simulink model "AION_IDS_SPEEDGOAT"  (R2021a)
settings: configuration reference "AION_IDS_Speedgoat" (kept outside this file)
undefined symbols (not defined in the file): ADCU_SCU_CYCLE_TIME, AutoTrqWhlReq_test, BeamReq_test, BodyCtrlReq_test, BrakeReq_test, C, CONTROL_CYCLE_TIME, GearLvlReq_test, GearLvlReqVD_test, HornRingReq_test, LatCtrlReq_test, LngCtrlReq_test, SCU_ADCU_CYCLE_TIME, SteerAngReq_test, SteerWhlTorqReq_test, TurnLightReq_test
libraries: canmsglib x21, speedgoatlib_IO612 x8, simulink x1
(part 1 of 2)
settings Model: DataDictionary=AION_IDS.sldd  SimulationMode=external  ExtModeBatchMode=on  ExtModeTrigType=signal  Creator=xinrui  LastModifiedBy=Administrator
settings ConfigSetRef: SourceName=AION_IDS_Speedgoat

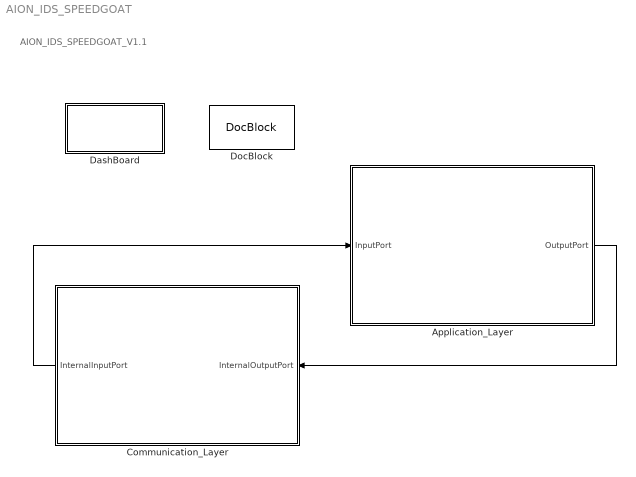
== system AION_IDS_SPEEDGOAT ==
  note: AION_IDS_SPEEDGOAT_V1.1
  Application_Layer : Subsystem
  Communication_Layer : Subsystem
  DashBoard : Subsystem
  DocBlock : simulink/Model-Wide Utilities/DocBlock  DocumentType=HTML  mask(DocBlock){}
      mask Display:
      | plot([.8 0 0 1 1 .8 .8 1],[1 1 0 0 .8 1 .8 .8]);
      | text(.5,.6,'CHANGELOG','horizontalalignment','center');
      | text(.95,.05,get_param(gcb,'DocumentType'),'verticalalignment','bottom','horizontalalignment','right');
  wires:
  Application_Layer/1(OutputPort) -> Communication_Layer/1(InternalOutputPort)
  Communication_Layer/1(InternalInputPort) -> Application_Layer/1(InputPort)

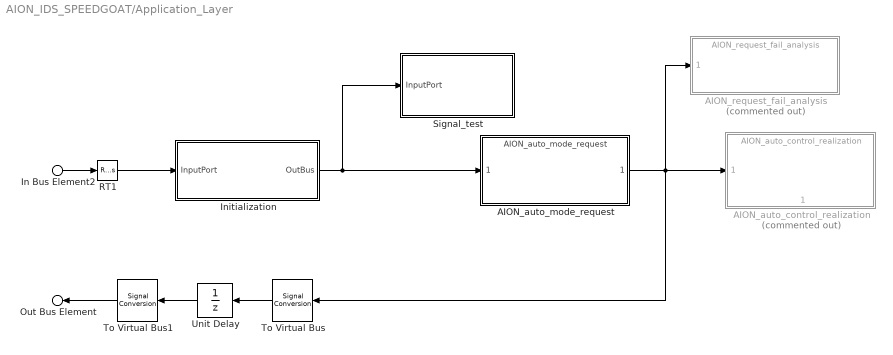
== system AION_IDS_SPEEDGOAT/Application_Layer ==
  In Bus Element2 : Inport  PortName=InputPort
  AION_auto_control_realization : ModelReference  Commented=on  ModelNameDialog=AION_auto_control_realization.slx  SimulationMode=Normal  ModelReferenceVersion=1.101
      settings: PortSchema="{\"entries\":[{\"content\":{\"sides\":[{\"content\":{\"connectorIds\":[\"In1\"]},\"type\":\"ConnectorPlacement.EquallySpacedRectSide\",\"uuid\":\"f3babb6e-c9bf-4030-9d63-e22104215124\"},{\"content\":{\"connectorIds\":[],\"side\":\"RIGHT\"},\"type\":\"ConnectorPlacement.EquallySpacedRectSide\",\"uuid\":\"12e9a174-2d38-44c0-9805-ab206046c590\"},{\"content\":{\"connectorIds\":[],\"side\":\"TOP\"},\"type\":\"ConnectorPlacement.EquallySpacedRectSide\",\"uuid\":\"6d900b41-a39b-4f3d-8ade-bd92ea251a29\"},{\"content\":{\"connectorIds\":[\"Out1\"],\"side\":\"BOTTOM\"},\"type\":\"ConnectorPlacement.EquallySpacedRectSide\",\"uuid\":\"aec3e921-60a7-468b-aade-685da2e04e8e\"}]},\"type\":\"ConnectorPlacement.EquallySpacedConnector\",\"uuid\":\"2f59d3d1-446e-4d33-80ca-cc7645fc2f83\"}],\"packageUris\":[\"http://schema.mathworks.com/mf0/Connector/R2020b\"],\"version\":\"1.0\"}"
  AION_auto_mode_request : ModelReference  ModelNameDialog=AION_auto_mode_request.slx  SimulationMode=Normal  ModelReferenceVersion=1.93
  AION_request_fail_analysis : ModelReference  Commented=on  ModelNameDialog=AION_request_fail_analysis.slx  SimulationMode=Normal  ModelReferenceVersion=1.33
  Initialization : Subsystem
  RT1 : RateTransition  Deterministic=off  OutPortSampleTimeOpt=Inherit
  Signal_test : Subsystem
  To Virtual Bus : SignalConversion  ConversionOutput=Nonvirtual bus  OutDataTypeStr=Bus: AION_ApplicationBus  OverrideOpt=off
  To Virtual Bus1 : SignalConversion  ConversionOutput=Virtual bus  OverrideOpt=off
  Unit Delay : UnitDelay  SampleTime=CONTROL_CYCLE_TIME  HasFrameUpgradeWarning=on
  Out Bus Element : Outport  PortName=OutputPort
  wires:
  To Virtual Bus/1 -> Unit Delay/1
  Unit Delay/1 -> To Virtual Bus1/1
  To Virtual Bus1/1 -> Out Bus Element/1
  AION_auto_mode_request/1 -> To Virtual Bus/1, AION_auto_control_realization/1, AION_request_fail_analysis/1
  In Bus Element2/1 -> RT1/1
  RT1/1 -> Initialization/1(InputPort)
  Initialization/1(OutBus) -> AION_auto_mode_request/1, Signal_test/1(InputPort)

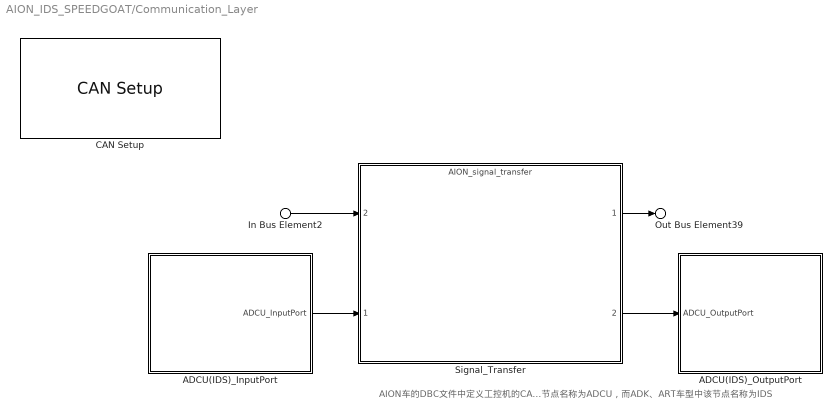
== system AION_IDS_SPEEDGOAT/Communication_Layer ==
  note: AION车的DBC文件中定义工控机的CAN节点名称为ADCU，而ADK、ART车型中该节点名称为IDS
  In Bus Element2 : Inport  PortName=InternalOutputPort
  ADCU(IDS)_InputPort : Subsystem
  ADCU(IDS)_OutputPort : Subsystem
  CAN Setup : speedgoatlib_IO612/CAN Setup  id=1  drvLtr=C:  PCISlot=-1  port1=CAN (HS)  port2=CAN (HS)  port3=Disable  port4=Disable  opModeCAN1=Highspeed (HS)  bdrCAN1=500 kBaud  usrBdrCAN1=[10, 1, 13, 2]  stdAccMaskCAN1=[0, 0]  extAccMaskCAN1=[0, 0]  opModeCAN2=Highspeed (HS)  bdrCAN2=500 kBaud  usrBdrCAN2=[10, 1, 13, 2]  stdAccMaskCAN2=[0, 0]  extAccMaskCAN2=[0, 0]  opModeCAN3=Highspeed (HS)  bdrCAN3=500 kBaud  usrBdrCAN3=[10, 1, 13, 2]  stdAccMaskCAN3=[0, 0]  extAccMaskCAN3=[0, 0]  opModeCAN4=Highspeed (HS)  bdrCAN4=500 kBaud  usrBdrCAN4=[10, 1, 13, 2]  stdAccMaskCAN4=[0, 0]  extAccMaskCAN4=[0, 0]  initStruct=[]  termStruct=[]  protl=IO612  qtyMod=1  chNo=[1, 2, 3, 4]  ptTypes=[1, 1, 1, 1]  protlHelpIdx=[0, 1, 2, 3]  isFDMod=0
      settings: SourceProductName=Simulink Real-Time: Speedgoat Library
  Signal_Transfer : ModelReference  ModelNameDialog=AION_signal_transfer.slx  SimulationMode=Normal  ModelReferenceVersion=4.81
      settings: PortSchema="{\"entries\":[{\"content\":{\"sides\":[{\"content\":{\"connectorIds\":[\"In2\",\"In1\"]},\"type\":\"ConnectorPlacement.EquallySpacedRectSide\",\"uuid\":\"d7b49387-9132-4f68-80a0-6c78bc11624f\"},{\"content\":{\"connectorIds\":[\"Out1\",\"Out2\"],\"side\":\"RIGHT\"},\"type\":\"ConnectorPlacement.EquallySpacedRectSide\",\"uuid\":\"3b80b3bd-44fe-4064-8909-e0d3ddc33b1d\"},{\"content\":{\"connectorIds\":[],\"side\":\"TOP\"},\"type\":\"ConnectorPlacement.EquallySpacedRectSide\",\"uuid\":\"9e6df871-f0e1-4d71-be51-8adc92933544\"}]},\"type\":\"ConnectorPlacement.EquallySpacedConnector\",\"uuid\":\"d7e504ac-b336-4965-bcb2-373027d2eba4\"}],\"packageUris\":[\"http://schema.mathworks.com/mf0/Connector/R2020b\"],\"version\":\"1.0\"}"
  Out Bus Element39 : Outport  PortName=InternalInputPort
  wires:
  Signal_Transfer/2 -> ADCU(IDS)_OutputPort/1(ADCU_OutputPort)
  In Bus Element2/1 -> Signal_Transfer/2
  ADCU(IDS)_InputPort/1(ADCU_InputPort) -> Signal_Transfer/1
  Signal_Transfer/1 -> Out Bus Element39/1

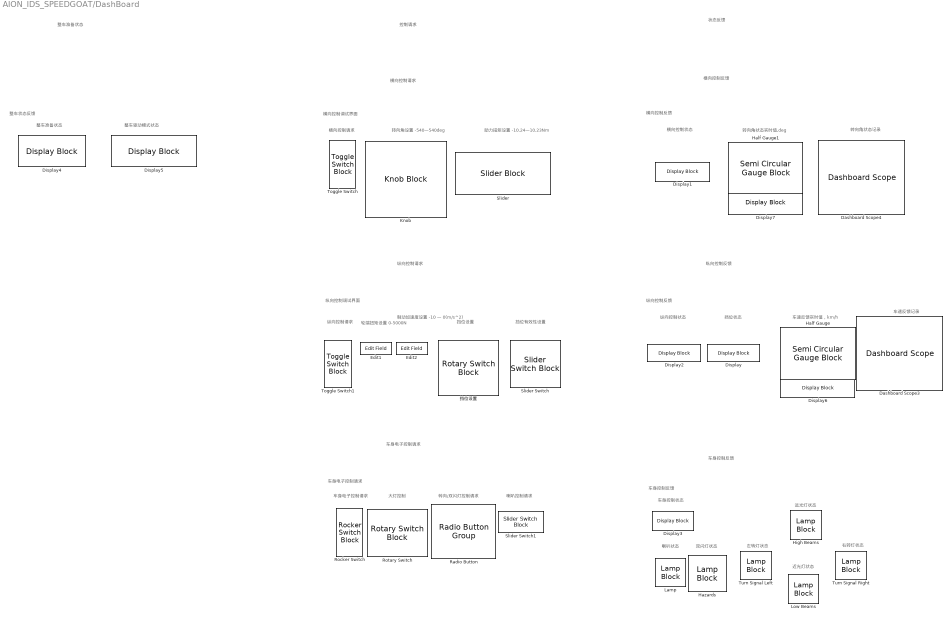
== system AION_IDS_SPEEDGOAT/DashBoard ==
  note: 纵向控制调试界面
  note: 横向控制调试界面
  note: 横向控制请求
  note: 纵向控制请求
  note: 挡位设置
  note: 挡位有效性设置
  note: 轮端扭矩设置
      | 0-5000N
  note: 制动加速度设置
      | -10 — 0(m/s^2)
  note: 转向角设置
      | -540—540deg
  note: 助力扭矩设置
      | -10.24—10.23Nm
  note: 车身电子控制请求
  note: 整车状态反馈
  note: 车身电子控制请求
  note: 车身电子控制请求
  note: 纵向控制请求
  note: 横向控制请求
  note: 纵向控制反馈
  note: 大灯控制
  note: 转向/双闪灯控制请求
  note: 喇叭控制请求
  note: 控制请求
  note: 状态反馈
  note: 横向控制反馈
  note: 横向控制反馈
  note: 车身控制反馈
  note: 车身控制反馈
  note: 车速反馈实时值，km/h
  note: 纵向控制状态
  note: 挡位状态
  note: 横向控制状态
  note: 转向角状态实时值,deg
  note: 转向角状态记录
  note: 车速反馈记录
  note: 喇叭状态
  note: 左转灯状态
  note: 远光灯状态
  note: 右转灯状态
  note: 双闪灯状态
  note: 车身控制状态
  note: 近光灯状态
  note: 纵向控制反馈
  note: 整车准备状态
  note: 整车准备状态
  note: 整车驱动模式状态
  Dashboard Scope3 : DashboardScope  Ymin=0  Ymax=130
  Dashboard Scope4 : DashboardScope  Ymin=-480  Ymax=480
  Display{,1..7} (8 alike) : DisplayBlock  LabelPosition=Hide  Format=short  Transparency=1
  Edit1 : EditField  LabelPosition=Hide  ShowInitialText=on  Alignment=Center
  Edit2 : EditField  LabelPosition=Hide  ShowInitialText=on  Alignment=Center
  Half Gauge : SemiCircularGaugeBlock  ScaleMax=150
  Half Gauge1 : SemiCircularGaugeBlock  ScaleMin=-480  ScaleMax=480
  Hazards : LampBlock  Icon=Hazards
  High Beams : LampBlock  Icon=HighBeams
  Knob : KnobBlock  ScaleMin=-540  ScaleMax=540
  Lamp : LampBlock
  Low Beams : LampBlock  Icon=LowBeams
  Radio Button : RadioButtonGroup  SelectedLabel=No request  ButtonGroupName=Group
      settings: Values={{'No request', 'Turn left lig', 'Turn right light', 'Emergency light'}, [0 1 2 3]}
  Rocker Switch : RockerSwitchBlock
      settings: Values={{'Disable', 'Enable'}, [0 1]}
  Rotary Switch : RotarySwitchBlock
      settings: Values={{'OFF', 'Low', 'High'}, [0 1 2]}
  Slider : SliderBlock  ScaleMin=-10  ScaleMax=10
  Slider Switch : SliderSwitchBlock
      settings: Values={{'Valid', 'Invalid'}, [1 0]}
  Slider Switch1 : SliderSwitchBlock
      settings: Values={{'Active', 'No active'}, [1 0]}
  Toggle Switch : ToggleSwitchBlock
      settings: Values={{'Manual', 'Auto'}, [0 1]}
  Toggle Switch1 : ToggleSwitchBlock
      settings: Values={{'Manual', 'Auto'}, [0 1]}
  Turn Signal Left : LampBlock  Icon=TurnSignalLeft
  Turn Signal Right : LampBlock  Icon=TurnSignalRight
  挡位设置 : RotarySwitchBlock
      settings: Values={{'No request', 'Park', 'Reversed', 'Neutral', 'Drive'}, [0 1 2 3 4]}

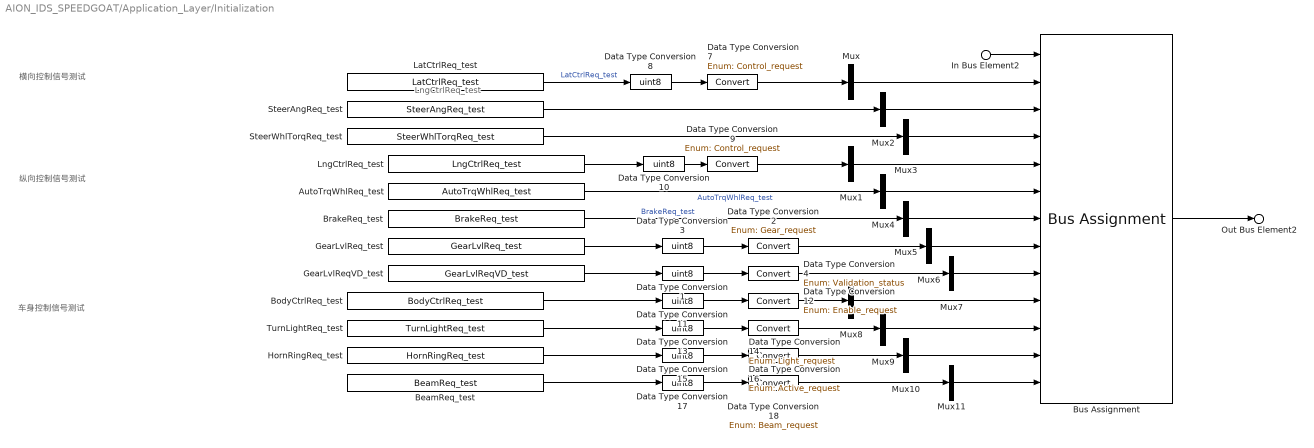
== system AION_IDS_SPEEDGOAT/Application_Layer/Initialization ==
  note: LngCtrlReq_test
  note: 横向控制信号测试
  note: 纵向控制信号测试
  note: 车身控制信号测试
  In Bus Element2 : Inport  PortName=InputPort
  AutoTrqWhlReq_test : Constant  Value=AutoTrqWhlReq_test  OutDataTypeStr=double  SampleTime=CONTROL_CYCLE_TIME
  BeamReq_test : Constant  Value=BeamReq_test  OutDataTypeStr=double  SampleTime=CONTROL_CYCLE_TIME
  BodyCtrlReq_test : Constant  Value=BodyCtrlReq_test  OutDataTypeStr=double  SampleTime=CONTROL_CYCLE_TIME
  BrakeReq_test : Constant  Value=BrakeReq_test  OutDataTypeStr=double  SampleTime=CONTROL_CYCLE_TIME
  Bus Assignment : BusAssignment  AssignedSignals=set_lateral_control_info.set_LatCtrlReq,set_lateral_control_info.set_SteerAngReq,set_lateral_control_info.set_SteerWhlTorqReq,set_longitudinal_control_info.set_LngCtrlReq,set_longitudinal_control_info.set_AutoTrqWhlReq,set_longitudinal_control_info.set_BrakeReq,set_longitudinal_control_info.set_GearLvlReq,set_longitudinal_control_info.set_GearLvlReqVD,set_ADCU_info.set_BodyCtrlReq,set_ADCU_info.set_TurnLightReq,set_ADCU_info.set_HornRingReq,set_ADCU_info.set_BeamReq
  Data Type Conversion{1,3,8,10..11,13,15,17} (8 alike) : DataTypeConversion  OutDataTypeStr=uint8
  Data Type Conversion12 : DataTypeConversion  OutDataTypeStr=Enum: Enable_request
  Data Type Conversion14 : DataTypeConversion  OutDataTypeStr=Enum: Light_request
  Data Type Conversion16 : DataTypeConversion  OutDataTypeStr=Enum: Active_request
  Data Type Conversion18 : DataTypeConversion  OutDataTypeStr=Enum: Beam_request
  Data Type Conversion2 : DataTypeConversion  OutDataTypeStr=Enum: Gear_request
  Data Type Conversion4 : DataTypeConversion  OutDataTypeStr=Enum: Validation_status
  Data Type Conversion7 : DataTypeConversion  OutDataTypeStr=Enum: Control_request
  Data Type Conversion9 : DataTypeConversion  OutDataTypeStr=Enum: Control_request
  GearLvlReqVD_test : Constant  Value=GearLvlReqVD_test  OutDataTypeStr=double  SampleTime=CONTROL_CYCLE_TIME
  GearLvlReq_test : Constant  Value=GearLvlReq_test  OutDataTypeStr=double  SampleTime=CONTROL_CYCLE_TIME
  HornRingReq_test : Constant  Value=HornRingReq_test  OutDataTypeStr=double  SampleTime=CONTROL_CYCLE_TIME
  LatCtrlReq_test : Constant  Value=LatCtrlReq_test  OutDataTypeStr=double  SampleTime=CONTROL_CYCLE_TIME
  LngCtrlReq_test : Constant  Value=LngCtrlReq_test  OutDataTypeStr=double  SampleTime=CONTROL_CYCLE_TIME
  Mux{,1..11} (12 alike) : Mux  Inputs=1
  SteerAngReq_test : Constant  Value=SteerAngReq_test  OutDataTypeStr=double  SampleTime=CONTROL_CYCLE_TIME
  SteerWhlTorqReq_test : Constant  Value=SteerWhlTorqReq_test  OutDataTypeStr=double  SampleTime=CONTROL_CYCLE_TIME
  TurnLightReq_test : Constant  Value=TurnLightReq_test  OutDataTypeStr=double  SampleTime=CONTROL_CYCLE_TIME
  Out Bus Element2 : Outport  PortName=OutBus
  wires:
  In Bus Element2/1 -> Bus Assignment/1
  Bus Assignment/1 -> Out Bus Element2/1
  Data Type Conversion9/1 -> Mux1/1
  Data Type Conversion10/1 -> Data Type Conversion9/1
  Data Type Conversion8/1 -> Data Type Conversion7/1
  Data Type Conversion7/1 -> Mux/1
  LngCtrlReq_test/1 -> Data Type Conversion10/1
  SteerWhlTorqReq_test/1 -> Mux3/1
  GearLvlReq_test/1 -> Data Type Conversion3/1
  SteerAngReq_test/1 -> Mux2/1
  AutoTrqWhlReq_test/1 -> Mux4/1  "AutoTrqWhlReq_test"
  Data Type Conversion1/1 -> Data Type Conversion4/1
  GearLvlReqVD_test/1 -> Data Type Conversion1/1
  Data Type Conversion3/1 -> Data Type Conversion2/1
  BrakeReq_test/1 -> Mux5/1  "BrakeReq_test"
  Data Type Conversion2/1 -> Mux6/1
  Data Type Conversion4/1 -> Mux7/1
  LatCtrlReq_test/1 -> Data Type Conversion8/1  "LatCtrlReq_test"
  Mux7/1 -> Bus Assignment/9
  Mux6/1 -> Bus Assignment/8
  Mux3/1 -> Bus Assignment/4
  Mux2/1 -> Bus Assignment/3
  Mux1/1 -> Bus Assignment/5
  Mux/1 -> Bus Assignment/2
  Data Type Conversion12/1 -> Mux8/1
  Data Type Conversion11/1 -> Data Type Conversion12/1
  Data Type Conversion13/1 -> Data Type Conversion14/1
  Data Type Conversion14/1 -> Mux9/1
  Data Type Conversion16/1 -> Mux10/1
  Data Type Conversion15/1 -> Data Type Conversion16/1
  Data Type Conversion17/1 -> Data Type Conversion18/1
  Data Type Conversion18/1 -> Mux11/1
  BodyCtrlReq_test/1 -> Data Type Conversion11/1
  TurnLightReq_test/1 -> Data Type Conversion13/1
  HornRingReq_test/1 -> Data Type Conversion15/1
  BeamReq_test/1 -> Data Type Conversion17/1
  Mux11/1 -> Bus Assignment/13
  Mux10/1 -> Bus Assignment/12
  Mux9/1 -> Bus Assignment/11
  Mux8/1 -> Bus Assignment/10
  Mux4/1 -> Bus Assignment/6
  Mux5/1 -> Bus Assignment/7

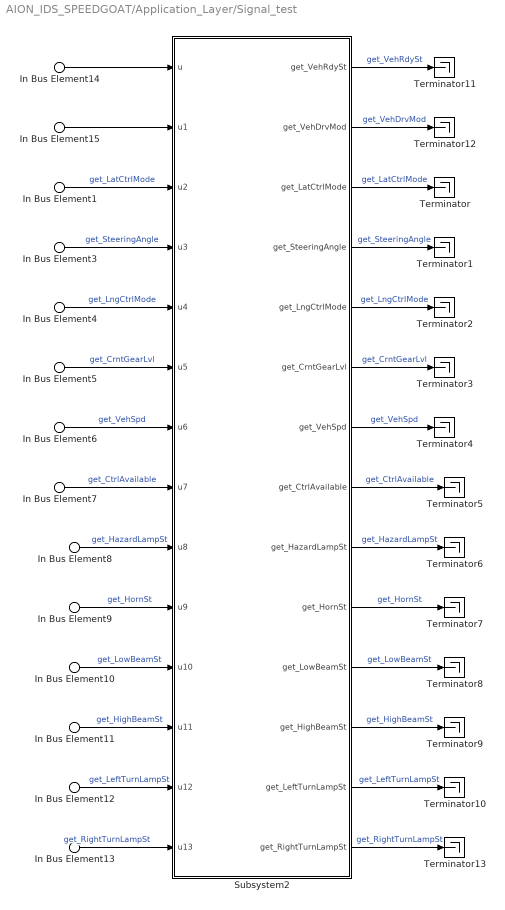
== system AION_IDS_SPEEDGOAT/Application_Layer/Signal_test ==
  In Bus Element6 : Inport  PortName=InputPort  Element=get_BCS_info.get_VehSpd
  In Bus Element15 : Inport  PortName=InputPort  Element=get_VCU_info.get_VehDrvMod
  In Bus Element14 : Inport  PortName=InputPort  Element=get_VCU_info.get_VehRdySt
  In Bus Element5 : Inport  PortName=InputPort  Element=get_VCU_info.get_CrntGearLvl
  In Bus Element1 : Inport  PortName=InputPort  Element=get_SCU_info.get_LatCtrlMode
  In Bus Element4 : Inport  PortName=InputPort  Element=get_SCU_info.get_LngCtrlMode
  In Bus Element3 : Inport  PortName=InputPort  Element=get_EPS_info.get_SteeringAngle
  In Bus Element7 : Inport  PortName=InputPort  Element=get_BCM_info.get_CtrlAvailable
  In Bus Element8 : Inport  PortName=InputPort  Element=get_BCM_info.get_HazardLampSt
  In Bus Element11 : Inport  PortName=InputPort  Element=get_BCM_info.get_HighBeamSt
  In Bus Element9 : Inport  PortName=InputPort  Element=get_BCM_info.get_HornSt
  In Bus Element12 : Inport  PortName=InputPort  Element=get_BCM_info.get_LeftTurnLampSt
  In Bus Element10 : Inport  PortName=InputPort  Element=get_BCM_info.get_LowBeamSt
  In Bus Element13 : Inport  PortName=InputPort  Element=get_BCM_info.get_RightTurnLampSt
  Subsystem2 : Subsystem
  Terminator{,1..13} (14 alike) : Terminator
  wires:
  In Bus Element14/1 -> Subsystem2/1(u)
  Subsystem2/1(get_VehRdySt) -> Terminator11/1  "get_VehRdySt"
  In Bus Element15/1 -> Subsystem2/2(u1)
  Subsystem2/3(get_LatCtrlMode) -> Terminator/1  "get_LatCtrlMode"
  Subsystem2/4(get_SteeringAngle) -> Terminator1/1  "get_SteeringAngle"
  Subsystem2/5(get_LngCtrlMode) -> Terminator2/1  "get_LngCtrlMode"
  Subsystem2/11(get_LowBeamSt) -> Terminator8/1  "get_LowBeamSt"
  Subsystem2/2(get_VehDrvMod) -> Terminator12/1  "get_VehDrvMod"
  Subsystem2/10(get_HornSt) -> Terminator7/1  "get_HornSt"
  Subsystem2/12(get_HighBeamSt) -> Terminator9/1  "get_HighBeamSt"
  Subsystem2/6(get_CrntGearLvl) -> Terminator3/1  "get_CrntGearLvl"
  Subsystem2/9(get_HazardLampSt) -> Terminator6/1  "get_HazardLampSt"
  Subsystem2/13(get_LeftTurnLampSt) -> Terminator10/1  "get_LeftTurnLampSt"
  Subsystem2/8(get_CtrlAvailable) -> Terminator5/1  "get_CtrlAvailable"
  Subsystem2/7(get_VehSpd) -> Terminator4/1  "get_VehSpd"
  Subsystem2/14(get_RightTurnLampSt) -> Terminator13/1  "get_RightTurnLampSt"
  In Bus Element8/1 -> Subsystem2/9(u8)  "get_HazardLampSt"
  In Bus Element9/1 -> Subsystem2/10(u9)  "get_HornSt"
  In Bus Element10/1 -> Subsystem2/11(u10)  "get_LowBeamSt"
  In Bus Element11/1 -> Subsystem2/12(u11)  "get_HighBeamSt"
  In Bus Element12/1 -> Subsystem2/13(u12)  "get_LeftTurnLampSt"
  In Bus Element13/1 -> Subsystem2/14(u13)  "get_RightTurnLampSt"
  In Bus Element1/1 -> Subsystem2/3(u2)  "get_LatCtrlMode"
  In Bus Element3/1 -> Subsystem2/4(u3)  "get_SteeringAngle"
  In Bus Element4/1 -> Subsystem2/5(u4)  "get_LngCtrlMode"
  In Bus Element5/1 -> Subsystem2/6(u5)  "get_CrntGearLvl"
  In Bus Element6/1 -> Subsystem2/7(u6)  "get_VehSpd"
  In Bus Element7/1 -> Subsystem2/8(u7)  "get_CtrlAvailable"

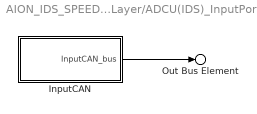
== system AION_IDS_SPEEDGOAT/Communication_Layer/ADCU(IDS)_InputPort ==
  InputCAN : Subsystem
  Out Bus Element : Outport  PortName=ADCU_InputPort  Element=InputCAN_bus
  wires:
  InputCAN/1(InputCAN_bus) -> Out Bus Element/1

== system AION_IDS_SPEEDGOAT/Communication_Layer/ADCU(IDS)_OutputPort ==
  Bus Element In : Inport  PortName=ADCU_OutputPort  Element=OutputCAN_bus
  OutputCAN : Subsystem
  wires:
  Bus Element In/1 -> OutputCAN/1(OutputCAN_bus)

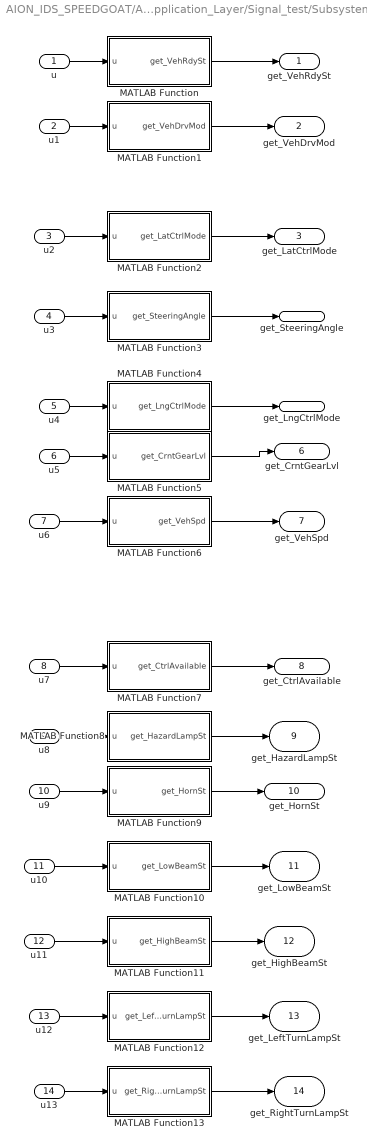
== system AION_IDS_SPEEDGOAT/Application_Layer/Signal_test/Subsystem2 ==
  u : Inport
  u1 : Inport  Port=2
  u2 : Inport  Port=3
  u3 : Inport  Port=4
  u4 : Inport  Port=5
  u5 : Inport  Port=6
  u6 : Inport  Port=7
  u7 : Inport  Port=8
  u8 : Inport  Port=9
  u9 : Inport  Port=10
  u10 : Inport  Port=11
  u11 : Inport  Port=12
  u12 : Inport  Port=13
  u13 : Inport  Port=14
  MATLAB Function : MATLAB Function  TreatAsAtomicUnit=on
  MATLAB Function1 : MATLAB Function  TreatAsAtomicUnit=on
  MATLAB Function10 : MATLAB Function  TreatAsAtomicUnit=on
  MATLAB Function11 : MATLAB Function  TreatAsAtomicUnit=on
  MATLAB Function12 : MATLAB Function  TreatAsAtomicUnit=on
  MATLAB Function13 : MATLAB Function  TreatAsAtomicUnit=on
  MATLAB Function2 : MATLAB Function  TreatAsAtomicUnit=on
  MATLAB Function3 : MATLAB Function  TreatAsAtomicUnit=on
  MATLAB Function4 : MATLAB Function  TreatAsAtomicUnit=on
  MATLAB Function5 : MATLAB Function  TreatAsAtomicUnit=on
  MATLAB Function6 : MATLAB Function  TreatAsAtomicUnit=on
  MATLAB Function7 : MATLAB Function  TreatAsAtomicUnit=on
  MATLAB Function8 : MATLAB Function  TreatAsAtomicUnit=on
  MATLAB Function9 : MATLAB Function  TreatAsAtomicUnit=on
  get_VehRdySt : Outport
  get_VehDrvMod : Outport  Port=2
  get_LatCtrlMode : Outport  Port=3
  get_SteeringAngle : Outport  Port=4
  get_LngCtrlMode : Outport  Port=5
  get_CrntGearLvl : Outport  Port=6
  get_VehSpd : Outport  Port=7
  get_CtrlAvailable : Outport  Port=8
  get_HazardLampSt : Outport  Port=9
  get_HornSt : Outport  Port=10
  get_LowBeamSt : Outport  Port=11
  get_HighBeamSt : Outport  Port=12
  get_LeftTurnLampSt : Outport  Port=13
  get_RightTurnLampSt : Outport  Port=14
  wires:
  u/1 -> MATLAB Function/1(u)
  u1/1 -> MATLAB Function1/1(u)
  u3/1 -> MATLAB Function3/1(u)
  u2/1 -> MATLAB Function2/1(u)
  u5/1 -> MATLAB Function5/1(u)
  u4/1 -> MATLAB Function4/1(u)
  u6/1 -> MATLAB Function6/1(u)
  u7/1 -> MATLAB Function7/1(u)
  u9/1 -> MATLAB Function9/1(u)
  u8/1 -> MATLAB Function8/1(u)
  MATLAB Function12/1(get_LeftTurnLampSt) -> get_LeftTurnLampSt/1
  u10/1 -> MATLAB Function10/1(u)
  u11/1 -> MATLAB Function11/1(u)
  MATLAB Function13/1(get_RightTurnLampSt) -> get_RightTurnLampSt/1
  MATLAB Function/1(get_VehRdySt) -> get_VehRdySt/1
  MATLAB Function1/1(get_VehDrvMod) -> get_VehDrvMod/1
  MATLAB Function2/1(get_LatCtrlMode) -> get_LatCtrlMode/1
  MATLAB Function3/1(get_SteeringAngle) -> get_SteeringAngle/1
  MATLAB Function4/1(get_LngCtrlMode) -> get_LngCtrlMode/1
  MATLAB Function6/1(get_VehSpd) -> get_VehSpd/1
  MATLAB Function5/1(get_CrntGearLvl) -> get_CrntGearLvl/1
  MATLAB Function7/1(get_CtrlAvailable) -> get_CtrlAvailable/1
  MATLAB Function8/1(get_HazardLampSt) -> get_HazardLampSt/1
  MATLAB Function9/1(get_HornSt) -> get_HornSt/1
  MATLAB Function10/1(get_LowBeamSt) -> get_LowBeamSt/1
  MATLAB Function11/1(get_HighBeamSt) -> get_HighBeamSt/1
  u12/1 -> MATLAB Function12/1(u)
  u13/1 -> MATLAB Function13/1(u)

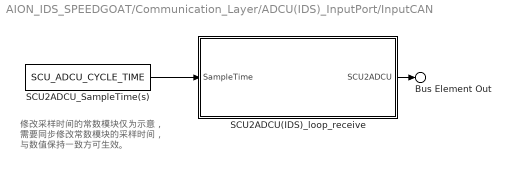
== system AION_IDS_SPEEDGOAT/Communication_Layer/ADCU(IDS)_InputPort/InputCAN ==
  note: 修改采样时间的常数模块仅为示意，
      | 需要同步修改常数模块的采样时间，
      | 与数值保持一致方可生效。
  SCU2ADCU(IDS)_loop_receive : Subsystem  TreatAsAtomicUnit=on
  SCU2ADCU_SampleTime(s) : Constant  Value=SCU_ADCU_CYCLE_TIME  SampleTime=ADCU_SCU_CYCLE_TIME
  Bus Element Out : Outport  PortName=InputCAN_bus  Element=SCU2ADCU_bus
  wires:
  SCU2ADCU_SampleTime(s)/1 -> SCU2ADCU(IDS)_loop_receive/1(SampleTime)
  SCU2ADCU(IDS)_loop_receive/1(SCU2ADCU) -> Bus Element Out/1

== system AION_IDS_SPEEDGOAT/Communication_Layer/ADCU(IDS)_OutputPort/OutputCAN ==
  Bus Element In : Inport  PortName=OutputCAN_bus  Element=ADCU2SCU_bus
  CAN_pack_ADCU2SCU : Subsystem
  wires:
  Bus Element In/1 -> CAN_pack_ADCU2SCU/1(ADCU2SCU)

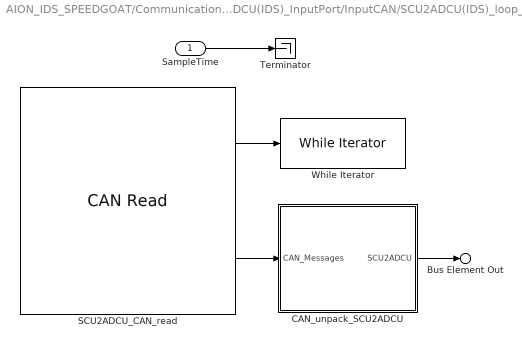
== system AION_IDS_SPEEDGOAT/Communication_Layer/ADCU(IDS)_InputPort/InputCAN/SCU2ADCU(IDS)_loop_receive ==
  SampleTime : Inport
  CAN_unpack_SCU2ADCU : Subsystem
  SCU2ADCU_CAN_read : speedgoatlib_IO612/CAN Read  id=1  sampleTime=-1  portSelection=1  messageType=CAN  protl=IO612  ptIdx=0  isFDMod=0
      settings: SourceProductName=Simulink Real-Time: Speedgoat Library
  Terminator : Terminator
  While Iterator : WhileIterator  MaxIters=-1  WhileBlockType=do-while
  Bus Element Out : Outport  PortName=SCU2ADCU
  wires:
  SCU2ADCU_CAN_read/1 -> While Iterator/1
  CAN_unpack_SCU2ADCU/1(SCU2ADCU) -> Bus Element Out/1
  SCU2ADCU_CAN_read/2 -> CAN_unpack_SCU2ADCU/1(CAN_Messages)
  SampleTime/1 -> Terminator/1

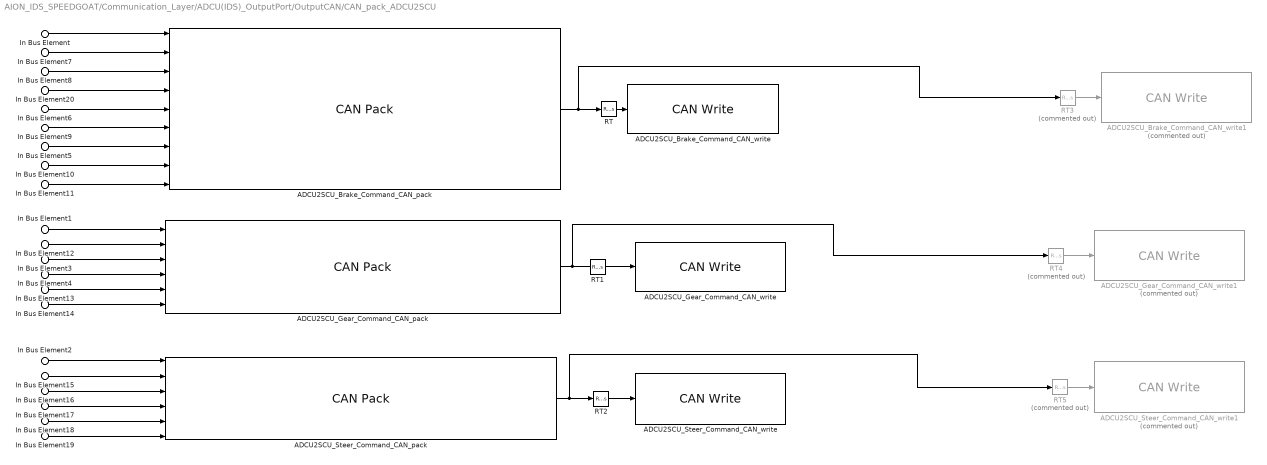
== system AION_IDS_SPEEDGOAT/Communication_Layer/ADCU(IDS)_OutputPort/OutputCAN/CAN_pack_ADCU2SCU ==
  In Bus Element : Inport  PortName=ADCU2SCU  Element=ADCU_1.ADCU_1_Checksum
  In Bus Element7 : Inport  PortName=ADCU2SCU  Element=ADCU_1.ADCU_1_MsgCounter
  In Bus Element8 : Inport  PortName=ADCU2SCU  Element=ADCU_1.ADCU_AutoTrqWhlReq
  In Bus Element20 : Inport  PortName=ADCU2SCU  Element=ADCU_1.ADCU_BrakeReq
  In Bus Element6 : Inport  PortName=ADCU2SCU  Element=ADCU_1.ADCU_GearLvlReq
  In Bus Element9 : Inport  PortName=ADCU2SCU  Element=ADCU_1.ADCU_GearLvlReqVD
  In Bus Element5 : Inport  PortName=ADCU2SCU  Element=ADCU_1.ADCU_LngCtrlReq
  In Bus Element10 : Inport  PortName=ADCU2SCU  Element=ADCU_1.ADCU_ParkingReqToEPB
  In Bus Element11 : Inport  PortName=ADCU2SCU  Element=ADCU_1.ADCU_ParkingReqToEPBVD
  In Bus Element1 : Inport  PortName=ADCU2SCU  Element=ADCU_2.ADCU_2_Checksum
  In Bus Element12 : Inport  PortName=ADCU2SCU  Element=ADCU_2.ADCU_2_MsgCounter
  In Bus Element3 : Inport  PortName=ADCU2SCU  Element=ADCU_2.ADCU_LatCtrlReq
  In Bus Element4 : Inport  PortName=ADCU2SCU  Element=ADCU_2.ADCU_SteerAngReq
  In Bus Element13 : Inport  PortName=ADCU2SCU  Element=ADCU_2.ADCU_SteerAngSpdLimt
  In Bus Element14 : Inport  PortName=ADCU2SCU  Element=ADCU_2.ADCU_SteerWhlTorqReq
  In Bus Element2 : Inport  PortName=ADCU2SCU  Element=ADCU_3.ADCU_3_Checksum
  In Bus Element15 : Inport  PortName=ADCU2SCU  Element=ADCU_3.ADCU_3_MsgCounter
  In Bus Element16 : Inport  PortName=ADCU2SCU  Element=ADCU_3.ADCU_BeamReq
  In Bus Element17 : Inport  PortName=ADCU2SCU  Element=ADCU_3.ADCU_BodyCtrlReq
  In Bus Element18 : Inport  PortName=ADCU2SCU  Element=ADCU_3.ADCU_HornRingReq
  In Bus Element19 : Inport  PortName=ADCU2SCU  Element=ADCU_3.ADCU_TurnLightReq
  ADCU2SCU_Brake_Command_CAN_pack : canmsglib/CAN Pack  CANdbFile=data\DBC\AION_ADCU_LX_L4_V1.6.1_210531.dbc  MsgList=ADCU_1  MsgName=ADCU_1  MsgIDType=Standard (11-bit identifier)  MsgIdentifier=544  MsgLength=8  Remote=off  ApplyMinMax=off  BusOutput=off  SignalInfo={'ADCU_1_Checksum','56','8','BE','unsigned','Standard','0','1','0','0','255';'ADCU_1_MsgCounter','48','4','BE','unsigned','Standard','0','1','0','0','15';'ADCU_AutoTrqWhlReq','26','14','BE','unsigned','Standard','0','1','-5000','-5000','5000';'ADCU_BrakeReq','8','16','BE','unsigned','Standard','0','0.0004882','-16','-16','16';'ADCU_GearLvlReq','37','3','BE','unsigned','Standard','0','1','0','0','7';'ADCU_GearLvlReqVD','36','1','BE','unsigned','Standard','0','1','0','0','1';'ADCU_LngCtrlReq','24','2','BE','unsigned','Standard','0','1','0','0','3';'ADCU_ParkingReqToEPB','35','1','BE','unsigned','Standard','0','1','0','0','1';'ADCU_ParkingReqToEPBVD','34','1','BE','unsigned','Standard','0','1','0','0','1'}
      settings: SourceProductBaseCode=ME,XP,VN  DataFormat=CANdb specified signals
  ADCU2SCU_Brake_Command_CAN_write : speedgoatlib_IO612/CAN Write  id=1  sampleTime=ADCU_SCU_CYCLE_TIME  portSelection=1  messageType=CAN  enaStatusPort=off  protl=IO612  ptIdx=0  isFDMod=0
      settings: SourceProductName=Simulink Real-Time: Speedgoat Library
  ADCU2SCU_Brake_Command_CAN_write1 : speedgoatlib_IO612/CAN Write  Commented=on  id=1  sampleTime=ADCU_SCU_CYCLE_TIME  portSelection=2  messageType=CAN  enaStatusPort=off  protl=IO612  ptIdx=1  isFDMod=0
      settings: SourceProductName=Simulink Real-Time: Speedgoat Library
  ADCU2SCU_Gear_Command_CAN_pack : canmsglib/CAN Pack  CANdbFile=data\DBC\AION_ADCU_LX_L4_V1.6.1_210531.dbc  MsgList=ADCU_2  MsgName=ADCU_2  MsgIDType=Standard (11-bit identifier)  MsgIdentifier=545  MsgLength=8  Remote=off  ApplyMinMax=off  BusOutput=off  SignalInfo={'ADCU_2_Checksum','56','8','BE','unsigned','Standard','0','1','0','0','255';'ADCU_2_MsgCounter','48','4','BE','unsigned','Standard','0','1','0','0','15';'ADCU_LatCtrlReq','44','1','BE','unsigned','Standard','0','1','0','0','1';'ADCU_SteerAngReq','8','16','BE','unsigned','Standard','0','0.1','-780','-780','779.9';'ADCU_SteerAngSpdLimt','24','16','BE','unsigned','Standard','0','0.125','0','0','1080';'ADCU_SteerWhlTorqReq','45','11','BE','unsigned','Standard','0','0.01','-10.24','-10.24','10.23'}
      settings: SourceProductBaseCode=ME,XP,VN  DataFormat=CANdb specified signals
  ADCU2SCU_Gear_Command_CAN_write : speedgoatlib_IO612/CAN Write  id=1  sampleTime=ADCU_SCU_CYCLE_TIME  portSelection=1  messageType=CAN  enaStatusPort=off  protl=IO612  ptIdx=0  isFDMod=0
      settings: SourceProductName=Simulink Real-Time: Speedgoat Library
  ADCU2SCU_Gear_Command_CAN_write1 : speedgoatlib_IO612/CAN Write  Commented=on  id=1  sampleTime=ADCU_SCU_CYCLE_TIME  portSelection=2  messageType=CAN  enaStatusPort=off  protl=IO612  ptIdx=1  isFDMod=0
      settings: SourceProductName=Simulink Real-Time: Speedgoat Library
  ADCU2SCU_Steer_Command_CAN_pack : canmsglib/CAN Pack  CANdbFile=data\DBC\AION_ADCU_LX_L4_V1.6.1_210531.dbc  MsgList=ADCU_3  MsgName=ADCU_3  MsgIDType=Standard (11-bit identifier)  MsgIdentifier=640  MsgLength=8  Remote=off  ApplyMinMax=off  BusOutput=off  SignalInfo={'ADCU_3_Checksum','56','8','BE','unsigned','Standard','0','1','0','0','255';'ADCU_3_MsgCounter','48','4','BE','unsigned','Standard','0','1','0','0','15';'ADCU_BeamReq','2','2','BE','unsigned','Standard','0','1','0','0','3';'ADCU_BodyCtrlReq','4','1','BE','unsigned','Standard','0','1','0','0','1';'ADCU_HornRingReq','5','1','BE','unsigned','Standard','0','1','0','0','1';'ADCU_TurnLightReq','0','2','BE','unsigned','Standard','0','1','0','0','3'}
      settings: SourceProductBaseCode=ME,XP,VN  DataFormat=CANdb specified signals
  ADCU2SCU_Steer_Command_CAN_write : speedgoatlib_IO612/CAN Write  id=1  sampleTime=ADCU3_SCU_CYCLE_TIME  portSelection=1  messageType=CAN  enaStatusPort=off  protl=IO612  ptIdx=0  isFDMod=0
      settings: SourceProductName=Simulink Real-Time: Speedgoat Library
  ADCU2SCU_Steer_Command_CAN_write1 : speedgoatlib_IO612/CAN Write  Commented=on  id=1  sampleTime=ADCU3_SCU_CYCLE_TIME  portSelection=2  messageType=CAN  enaStatusPort=off  protl=IO612  ptIdx=1  isFDMod=0
      settings: SourceProductName=Simulink Real-Time: Speedgoat Library
  RT : RateTransition  Deterministic=off  OutPortSampleTime=0.02
  RT1 : RateTransition  Deterministic=off  OutPortSampleTime=0.02
  RT2 : RateTransition  Deterministic=off  OutPortSampleTime=0.05
  RT3 : RateTransition  Commented=on  Deterministic=off  OutPortSampleTime=0.02
  RT4 : RateTransition  Commented=on  Deterministic=off  OutPortSampleTime=0.02
  RT5 : RateTransition  Commented=on  Deterministic=off  OutPortSampleTime=0.05
  wires:
  In Bus Element1/1 -> ADCU2SCU_Gear_Command_CAN_pack/1
  In Bus Element2/1 -> ADCU2SCU_Steer_Command_CAN_pack/1
  In Bus Element4/1 -> ADCU2SCU_Gear_Command_CAN_pack/4
  In Bus Element3/1 -> ADCU2SCU_Gear_Command_CAN_pack/3
  In Bus Element13/1 -> ADCU2SCU_Gear_Command_CAN_pack/5
  In Bus Element12/1 -> ADCU2SCU_Gear_Command_CAN_pack/2
  In Bus Element14/1 -> ADCU2SCU_Gear_Command_CAN_pack/6
  In Bus Element15/1 -> ADCU2SCU_Steer_Command_CAN_pack/2
  In Bus Element16/1 -> ADCU2SCU_Steer_Command_CAN_pack/3
  In Bus Element17/1 -> ADCU2SCU_Steer_Command_CAN_pack/4
  In Bus Element18/1 -> ADCU2SCU_Steer_Command_CAN_pack/5
  In Bus Element19/1 -> ADCU2SCU_Steer_Command_CAN_pack/6
  In Bus Element11/1 -> ADCU2SCU_Brake_Command_CAN_pack/9
  In Bus Element10/1 -> ADCU2SCU_Brake_Command_CAN_pack/8
  In Bus Element5/1 -> ADCU2SCU_Brake_Command_CAN_pack/7
  In Bus Element/1 -> ADCU2SCU_Brake_Command_CAN_pack/1
  In Bus Element7/1 -> ADCU2SCU_Brake_Command_CAN_pack/2
  In Bus Element8/1 -> ADCU2SCU_Brake_Command_CAN_pack/3
  In Bus Element20/1 -> ADCU2SCU_Brake_Command_CAN_pack/4
  In Bus Element6/1 -> ADCU2SCU_Brake_Command_CAN_pack/5
  In Bus Element9/1 -> ADCU2SCU_Brake_Command_CAN_pack/6
  RT/1 -> ADCU2SCU_Brake_Command_CAN_write/1
  RT1/1 -> ADCU2SCU_Gear_Command_CAN_write/1
  RT2/1 -> ADCU2SCU_Steer_Command_CAN_write/1
  RT5/1 -> ADCU2SCU_Steer_Command_CAN_write1/1
  RT4/1 -> ADCU2SCU_Gear_Command_CAN_write1/1
  RT3/1 -> ADCU2SCU_Brake_Command_CAN_write1/1
  ADCU2SCU_Gear_Command_CAN_pack/1 -> RT4/1, RT1/1
  ADCU2SCU_Brake_Command_CAN_pack/1 -> RT3/1, RT/1
  ADCU2SCU_Steer_Command_CAN_pack/1 -> RT5/1, RT2/1
